simulink model "sine_kin"  (R2022a)
settings: Solver=VariableStepAuto  StartTime=0.0  StopTime=15  MaxStep=0.05  RelTol=1e-3
libraries: simulink x2
settings Model: Creator=patri  LastModifiedBy=Mattia
settings SolverCC: MaxConsecutiveMinStep=2  ShapePreserveControl=EnableAll

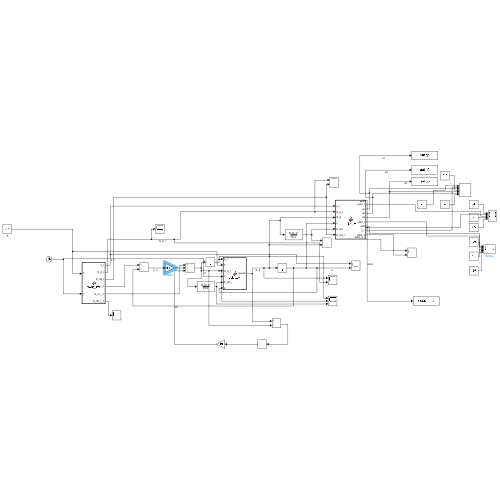
[thumbnail: Simulink's stored preview of the top-level diagram]
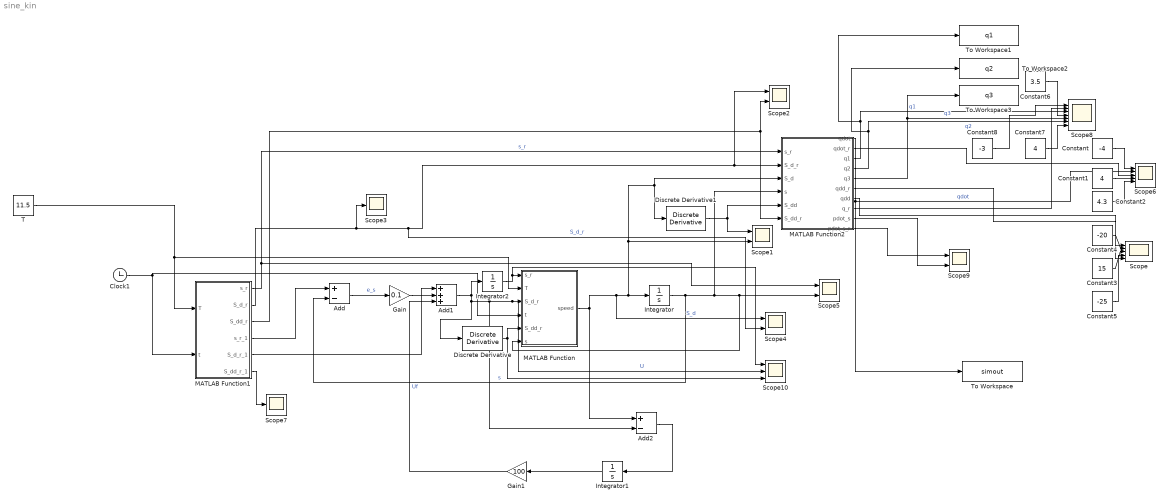
== system sine_kin ==
  Add : Sum  Inputs=+-
  Add1 : Sum  Inputs=+++
  Add2 : Sum  Inputs=+-
  Clock1 : Clock
  Constant : Constant  Value=-4
  Constant1 : Constant  Value=4
  Constant2 : Constant  Value=4.3
  Constant3 : Constant  Value=15
  Constant4 : Constant  Value=-20
  Constant5 : Constant  Value=-25
  Constant6 : Constant  Value=3.5
  Constant7 : Constant  Value=4
  Constant8 : Constant  Value=-3
  Discrete Derivative : simulink/Discrete/Discrete Derivative  gainval=1.0  ICPrevScaledInput=0.0  OutMin=[]  OutMax=[]  OutDataType=fixdt(1, 16)  OutScaling=2^-10  DoSatur=off
  Discrete Derivative1 : simulink/Discrete/Discrete Derivative  gainval=1.0  ICPrevScaledInput=0.0  OutMin=[]  OutMax=[]  OutDataType=fixdt(1, 16)  OutScaling=2^-10  DoSatur=off
  Gain : Gain  Gain=0.1
  Gain1 : Gain  Gain=100
  Integrator : Integrator
  Integrator1 : Integrator
  Integrator2 : Integrator
  MATLAB Function : MATLAB Function  TreatAsAtomicUnit=on
  MATLAB Function1 : MATLAB Function  TreatAsAtomicUnit=on
  MATLAB Function2 : MATLAB Function  TreatAsAtomicUnit=on
  Scope : Scope  NumInputPorts=5
  Scope{1..2,4..5,9} (5 alike) : Scope  NumInputPorts=2
  Scope10 : Scope  NumInputPorts=3
  Scope3 : Scope
  Scope6 : Scope  NumInputPorts=5
  Scope7 : Scope
  Scope8 : Scope  NumInputPorts=7
  T : Constant  Value=11.5
  To Workspace : ToWorkspace  VariableName=simout  SampleTime=-1
  To Workspace1 : ToWorkspace  VariableName=q1  SampleTime=-1
  To Workspace2 : ToWorkspace  VariableName=q2  SampleTime=-1
  To Workspace3 : ToWorkspace  VariableName=q3  SampleTime=-1
  wires:
  MATLAB Function1/1(s_r) -> MATLAB Function2/1(s_r), Scope5/1  "s_r"
  Add/1 -> Gain/1  "e_s"
  MATLAB Function1/2(S_d_r) -> Scope3/1, Scope4/2, Scope2/1, MATLAB Function2/2(S_d_r)  "S_d_r"
  Gain/1 -> Add1/2
  Add1/1 -> Discrete Derivative/1, Add2/2, Scope10/2, MATLAB Function/3(S_d_r), Integrator2/1  "U"
  MATLAB Function/1(speed) -> Scope4/1, Discrete Derivative1/1, MATLAB Function2/3(S_d), Scope1/2, Integrator/1, Add2/1  "S_d"
  Add2/1 -> Integrator1/1
  Integrator1/1 -> Gain1/1
  Gain1/1 -> Add1/3  "Uf"
  Integrator/1 -> Add/2, MATLAB Function2/4(s), MATLAB Function/6(s), Scope5/2  "s"
  Clock1/1 -> MATLAB Function1/2(t), MATLAB Function/4(t)
  MATLAB Function2/1(qdot) -> To Workspace/1, Scope6/2  "qdot"
  MATLAB Function2/2(qdot_r) -> Scope6/3
  MATLAB Function2/3(q1) -> To Workspace1/1, Scope8/3  "q1"
  MATLAB Function2/4(q2) -> To Workspace2/1, Scope8/6  "q2"
  MATLAB Function2/5(q3) -> To Workspace3/1, Scope8/5  "q3"
  T/1 -> MATLAB Function/2(T), MATLAB Function1/1(T)
  MATLAB Function2/6(qdd_r) -> Scope/1
  MATLAB Function2/7(qdd) -> Scope/5
  Constant/1 -> Scope6/1
  Constant1/1 -> Scope6/4
  Constant2/1 -> Scope6/5
  Constant5/1 -> Scope/4
  Constant3/1 -> Scope/3
  Discrete Derivative1/1 -> MATLAB Function2/5(S_dd), Scope1/1
  Constant4/1 -> Scope/2
  MATLAB Function1/3(S_dd_r) -> Scope2/2, MATLAB Function2/6(S_dd_r)
  MATLAB Function2/8(q_r) -> Scope8/2
  Constant6/1 -> Scope8/4
  Constant7/1 -> Scope8/7
  MATLAB Function2/9(pdot_s) -> Scope9/2
  MATLAB Function2/10(pdot_s_r) -> Scope9/1
  MATLAB Function1/4(s_r_1) -> Add/1
  MATLAB Function1/5(S_d_r_1) -> Add1/1
  MATLAB Function1/6(S_dd_r_1) -> Scope7/1
  Integrator2/1 -> Scope10/1, MATLAB Function/1(s_r)
  Discrete Derivative/1 -> Scope10/3, MATLAB Function/5(S_dd_r)
  Constant8/1 -> Scope8/1

== matlab function sine_kin/MATLAB Function ==
  data: s_r input; T input; speed output; S_d_r input; t input; S_dd_r input; s input
function speed = trajectory(s_r, T, S_d_r,t, S_dd_r, s)

%Links length
l1 = 1; l2 =1; l3 = 1;

%Trajectory


%%% REFERENCE


p_s_r =  [s_r + 1;
    1 + sin(4*pi*s_r);
    s_r];

R1_s_r=[1;
        4*pi*cos(4*pi*s_r);
        1];

%Velocity of the trajectory


%%pdot = R'*s'(t)




%%% REFERENCE

%%%POLYNOMIAL OF DEGREE 5 ---  0.4808 saturation --- 3.9 seconds
% pdot_s_r=[ -(30*t^2*pi*sin((2*t^3*pi*(10*T^2 - 15*T*t + 6*t^2))/T^5)*(T - t)^2)/T^5;
%           (30*t^2*pi*cos((2*t^3*pi*(10*T^2 - 15*T*t + 6*t^2))/T^5)*(T - t)^2)/T^5;
%                                                                                 0];
pdot_s_r= R1_s_r* S_d_r ; %sdr is u
      

%%%%%%%%%%%%%%%%%%%
% pdot_s_r = [-pi*sin(2*pi*((10*t^3)/T^3 - (15*t^4)/T^4 + (6*t^5)/T^5))*((30*t^2)/T^3 - (60*t^3)/T^4 + (30*t^4)/T^5);
%  pi*cos(2*pi*((10*t^3)/T^3 - (15*t^4)/T^4 + (6*t^5)/T^5))*((30*t^2)/T^3 - (60*t^3)/T^4 + (30*t^4)/T^5);
%                                                                                                      0];

%End effector position

%%% REFERENCE

px_r=p_s_r(1); py_r = p_s_r(2);
phi_r = p_s_r(3);

%%Inverse kinematics of planar 3R, compute q

%%% REFERENCE

p2_r = [px_r; py_r] - [l3*cos(phi_r); l3*sin(phi_r)];
p2x_r = p2_r(1);
p2y_r = p2_r(2);

% second joint computations


%%% REFERENCE

c2_r=(p2x_r^2+p2y_r^2-l1^2-l2^2)/(2*l1*l2); s2pos_r=sqrt(1-c2_r^2);

%other solution: -sqrt(1-c2^2)

%%% REFERENCE

s2neg_r=-sqrt(1-c2_r^2);

q02p_r=atan2(s2pos_r,c2_r);
q02n_r=atan2(s2neg_r,c2_r);
 
% first joint computations


%%% REFERENCE

detM_r=l1^2+l2^2+2*l1*l2*c2_r;

% positive solution of q1


%%% REFERENCE

s1pos_r=(p2y_r*(l1+l2*c2_r)-p2x_r*l2*s2pos_r)/detM_r; c1pos_r=(p2x_r*(l1+l2*c2_r)+p2y_r*l2*s2pos_r)/detM_r;

% negative solution of q1


%%% REFERENCE

s1neg_r=(p2y_r*(l1+l2*c2_r)-p2x_r*l2*s2neg_r)/detM_r;
c1neg_r=(p2x_r*(l1+l2*c2_r)+p2y_r*l2*s2neg_r)/detM_r;

q01p_r=atan2(s1pos_r,c1pos_r);
q01n_r=atan2(s1neg_r,c1neg_r); 

q03p_r = phi_r-(q01p_r+q02p_r);
q03n_r = phi_r-(q01n_r+q02n_r);



%%% REFERENCE


% output negative


%%% REFERENCE

q0n_r=[q01n_r; q02n_r; q03n_r];
q1_r = q0n_r(1);
q2_r = q0n_r(2);
q3_r = q0n_r(3);

%NOW WE COMPUTE qdot, qdotdot

%%% REFERENCE


P_r = [l1*cos(q1_r) + l2*cos(q1_r+q2_r) + l3*cos(q1_r+q2_r+q3_r);
    l1*sin(q1_r) + l2*sin(q1_r+q2_r) + l3*sin(q1_r+q2_r+q3_r)
    q1_r + q2_r + q3_r];

J_r = [- sin(q1_r + q2_r + q3_r) - sin(q1_r + q2_r) - sin(q1_r), - sin(q1_r + q2_r + q3_r) - sin(q1_r + q2_r), -sin(q1_r + q2_r + q3_r);
  cos(q1_r + q2_r + q3_r) + cos(q1_r + q2_r) + cos(q1_r),   cos(q1_r + q2_r + q3_r) + cos(q1_r + q2_r),  cos(q1_r + q2_r + q3_r);
                                          1,                                  1,                  1];


qdot_r = pinv(J_r) * pdot_s_r;

dq1_r=qdot_r(1);
dq2_r=qdot_r(2);
dq3_r=qdot_r(3);
J_dot_r = [- cos(q1_r + q2_r + q3_r)*(dq1_r + dq2_r + dq3_r) - cos(q1_r + q2_r)*(dq1_r + dq2_r) - dq1_r*cos(q1_r), - cos(q1_r + q2_r + q3_r)*(dq1_r + dq2_r + dq3_r) - cos(q1_r + q2_r)*(dq1_r + dq2_r), -cos(q1_r + q2_r + q3_r)*(dq1_r + dq2_r + dq3_r);
           - sin(q1_r + q2_r + q3_r)*(dq1_r + dq2_r + dq3_r) - sin(q1_r + q2_r)*(dq1_r + dq2_r) - dq1_r*sin(q1_r), - sin(q1_r + q2_r + q3_r)*(dq1_r + dq2_r + dq3_r) - sin(q1_r + q2_r)*(dq1_r + dq2_r), -sin(q1_r + q2_r + q3_r)*(dq1_r + dq2_r + dq3_r) ;   
            0,0,0];

%directly calculated
% pdd_r = [pi*sin(2*pi*((10*t^3)/T^3 - (15*t^4)/T^4 + (6*t^5)/T^5))*((60*t)/T^3 - (180*t^2)/T^4 + (120*t^3)/T^5) - 2*pi^2*cos(2*pi*((10*t^3)/T^3 - (15*t^4)/T^4 + (6*t^5)/T^5))*((30*t^2)/T^3 - (60*t^3)/T^4 + (30*t^4)/T^5)^2;
%        pi*cos(2*pi*((10*t^3)/T^3 - (15*t^4)/T^4 + (6*t^5)/T^5))*((60*t)/T^3 - (180*t^2)/T^4 + (120*t^3)/T^5) - 2*pi^2*sin(2*pi*((10*t^3)/T^3 - (15*t^4)/T^4 + (6*t^5)/T^5))*((30*t^2)/T^3 - (60*t^3)/T^4 + (30*t^4)/T^5)^2;
%         0];
 %%(60*t)/T^3 - (180*t^2)/T^4 + (120*t^3)/T^5

q1d_r=dq1_r;
q2d_r=dq2_r;
q3d_r=dq3_r;

pdotdot_s_r =[   0
        -16*pi^2*sin(4*pi*s_r)
                     0];

pdd_r = R1_s_r * S_dd_r + pdotdot_s_r * S_d_r^2;

qdd_r = inv(J_r)*(pdd_r - J_dot_r*qdot_r);

q1dd_r=qdd_r(1);
q2dd_r=qdd_r(2);
q3dd_r=qdd_r(3);
%%%%%%%%%%%%%%%%%%%%%%%%%%%%%%%%%%%%%%%%%%%%%%%%%%%%%%%%%%%%
%%bounds
q1_max=3.5;   q1_min=-3.5;
q2_max=3;     q2_min=-3;
q3_max= 2.57; q2_min =-2.57;
q1d_max= 4;   q1d_min=-4;
q2d_max=4;    q2d_min = -4;
q3d_max=4.3;  q3d_min=-4.3;
q1dd_max=20;  q1dd_min=-20;
q2dd_max=15;  q2dd_min=-15;
q3dd_max=20;  q3dd_min=-20;


constraint_pos = max([abs(q1_r/q1_max); abs(q2_r/q2_max);abs(q3_r/q3_max)]);

constraint_vel = max([abs(q1d_r/q1d_max);abs(q2d_r/q2d_max);abs(q3d_r/q3d_max)]);

constraint_acc = max([abs(q1dd_r/q1dd_max); abs(q2dd_r/q2dd_max);abs(q3dd_r/q3dd_max)]);

most_constrained = max([1;constraint_vel;(constraint_acc)]);

speed = S_d_r / most_constrained;

== matlab function sine_kin/MATLAB Function1 ==
  data: T input; t input; s_r output; S_d_r output; S_dd_r output; s_r_1 output; S_d_r_1 output; S_dd_r_1 output
function [s_r, S_d_r, S_dd_r,s_r_1, S_d_r_1, S_dd_r_1] = timing_law(T, t)
if t <T
    tau_t=t/T;
    %s_r = -2*tau_t^3 + 3*tau_t^2;
    %S_d_r=(6*t)/T^2 - (6*t^2)/T^3;
    s_r = 10*tau_t^3 - 15*tau_t^4 + 6*tau_t^5;
    S_d_r = (30*t^2)/T^3 - (60*t^3)/T^4 + (30*t^4)/T^5;
    S_dd_r = (60*t)/T^3 - (180*t^2)/T^4 + (120*t^3)/T^5;

    t_1 = t +0.0001;
    tau_t_1 = t_1/T;
    s_r_1 = 10*tau_t_1^3 - 15*tau_t_1^4 + 6*tau_t_1^5;
    S_d_r_1 = (30*t_1^2)/T^3 - (60*t_1^3)/T^4 + (30*t_1^4)/T^5;
    S_dd_r_1=(60*t_1)/T^3 - (180*t_1^2)/T^4 + (120*t_1^3)/T^5;

else 
    s_r = 1;
    S_d_r = 0;
    S_dd_r = 0;
    s_r_1 = 1;
    S_d_r_1 = 0;
    S_dd_r_1 = 0;
end

== matlab function sine_kin/MATLAB Function2 ==
  data: s_r input; S_d_r input; S_d input; s input; S_dd input; S_dd_r input; qdot output; qdot_r output; q1 output; q2 output; q3 output; qdd_r output; qdd output; q_r output; pdot_s output; pdot_s_r output
function [qdot,qdot_r,q1,q2,q3, qdd_r, qdd, q_r, pdot_s, pdot_s_r] = trajectory(s_r, S_d_r, S_d, s, S_dd, S_dd_r)

%Links length
l1 = 1; l2 =1; l3 = 1;

%Trajectory

p_s = [s + 1;
    1 + sin(4*pi*s);
    s];

p_s_r =  [s_r + 1;
    1 + sin(4*pi*s_r);
    s_r];

p1_s=[1;
        4*pi*cos(4*pi*s);
        1];
p1_s_r=[1;
        4*pi*cos(4*pi*s_r);
        1];

pdot_s= p1_s* S_d ;

                                                             
pdot_s_r = p1_s_r * S_d_r;
                                                             
                                                                    
%%%%%%%%%%%%%%%%%%%%%%%%%%%%%%%%%%%%%%%%%%%%%%%%%%%%%%%%%%%%%%%%
px = p_s(1); py = p_s(2); %position of the end effector w.r.t. the global frame

phi = p_s(3); %orientation of the end effector w.r.t. global frame

%%% REFERENCE

px_r=p_s_r(1); py_r = p_s_r(2);
phi_r = p_s_r(3);

%%Inverse kinematics of planar 3R
%fprintf("we first solve the joint variables q1, q2 in order to place\nthe position of the base of the third link in the necessary position\n");
 
p2 = [px; py] - [l3*cos(phi); l3*sin(phi)];
p2x = p2(1);
p2y = p2(2);

%%% REFERENCE

p2_r = [px_r; py_r] - [l3*cos(phi_r); l3*sin(phi_r)];
p2x_r = p2_r(1);
p2y_r = p2_r(2);

% second joint computations
c2=(p2x^2+p2y^2-l1^2-l2^2)/(2*l1*l2); 

%%% REFERENCE

c2_r=(p2x_r^2+p2y_r^2-l1^2-l2^2)/(2*l1*l2);

%other solution: -sqrt(1-c2^2)
s2neg=-sqrt(1-c2^2);


q02n=atan2(s2neg,c2);

%%% REFERENCE

s2neg_r=-sqrt(1-c2_r^2);


q02n_r=atan2(s2neg_r,c2_r);
 
% first joint computations
detM=l1^2+l2^2+2*l1*l2*c2;

%%% REFERENCE

detM_r=l1^2+l2^2+2*l1*l2*c2_r;


%%% REFERENCE



% negative solution of q1
s1neg=(p2y*(l1+l2*c2)-p2x*l2*s2neg)/detM;
c1neg=(p2x*(l1+l2*c2)+p2y*l2*s2neg)/detM;

q01n=atan2(s1neg,c1neg);
q03n = phi-(q01n+q02n);

%%% REFERENCE

s1neg_r=(p2y_r*(l1+l2*c2_r)-p2x_r*l2*s2neg_r)/detM_r;
c1neg_r=(p2x_r*(l1+l2*c2_r)+p2y_r*l2*s2neg_r)/detM_r;


q01n_r=atan2(s1neg_r,c1neg_r); 

q03n_r = phi_r-(q01n_r+q02n_r);


%%% REFERENCE


% output negative
q0n=[q01n; q02n; q03n];

%%% REFERENCE

q0n_r=[q01n_r; q02n_r; q03n_r];
q_r = q0n_r;
%In a cubic polynomial the maximum of the speed of the timing law is
%obtained in t = T/2 
q1 = q0n(1);
q2 = q0n(2);
q3 = q0n(3);
P = [l1*cos(q1) + l2*cos(q1+q2) + l3*cos(q1+q2+q3);
    l1*sin(q1) + l2*sin(q1+q2) + l3*sin(q1+q2+q3)
    q1 + q2 + q3];

J = [- sin(q1 + q2 + q3) - sin(q1 + q2) - sin(q1), - sin(q1 + q2 + q3) - sin(q1 + q2), -sin(q1 + q2 + q3);
  cos(q1 + q2 + q3) + cos(q1 + q2) + cos(q1),   cos(q1 + q2 + q3) + cos(q1 + q2),  cos(q1 + q2 + q3);
                                          1,                                  1,                  1];

%%% REFERENCE

q1_r = q0n_r(1);
q2_r = q0n_r(2);
q3_r = q0n_r(3);

P_r = [l1*cos(q1_r) + l2*cos(q1_r+q2_r) + l3*cos(q1_r+q2_r+q3_r);
    l1*sin(q1_r) + l2*sin(q1_r+q2_r) + l3*sin(q1_r+q2_r+q3_r)
    q1 + q2 + q3];

J_r = [- sin(q1_r + q2_r + q3_r) - sin(q1_r + q2_r) - sin(q1_r), - sin(q1_r + q2_r + q3_r) - sin(q1_r + q2_r), -sin(q1_r + q2_r + q3_r);
  cos(q1_r + q2_r + q3_r) + cos(q1_r + q2_r) + cos(q1_r),   cos(q1_r + q2_r + q3_r) + cos(q1_r + q2_r),  cos(q1_r + q2_r + q3_r);
                                          1,                                  1,                  1];


qdot = pinv(J) * pdot_s;
dq1 = qdot(1);
dq2 = qdot(2);
dq3 = qdot(3);

p2_s =[   0
-16*pi^2*sin(4*pi*s)
                     0];

J_dot = [- cos(q1 + q2 + q3)*(dq1 + dq2 + dq3) - cos(q1 + q2)*(dq1 + dq2) - dq1*cos(q1), - cos(q1 + q2 + q3)*(dq1 + dq2 + dq3) - cos(q1 + q2)*(dq1 + dq2), -cos(q1 + q2 + q3)*(dq1 + dq2 + dq3);
    - sin(q1 + q2 + q3)*(dq1 + dq2 + dq3) - sin(q1 + q2)*(dq1 + dq2) - dq1*sin(q1), - sin(q1 + q2 + q3)*(dq1 + dq2 + dq3) - sin(q1 + q2)*(dq1 + dq2), -sin(q1 + q2 + q3)*(dq1 + dq2 + dq3);
    0,0,0];
pdd = p1_s * S_dd + p2_s * S_d^2;
qdd = inv(J)*(pdd - J_dot*qdot);
%%% REFERENCE

qdot_r = pinv(J_r) * pdot_s_r;

qdot = qdot;
dq1_r = qdot_r(1); dq2_r = qdot_r(2); dq3_r = qdot_r(3);
qdot_r = qdot_r;
J_dot_r = [- cos(q1_r + q2_r + q3_r)*(dq1_r + dq2_r + dq3_r) - cos(q1_r + q2_r)*(dq1_r + dq2_r) - dq1_r*cos(q1_r), - cos(q1_r + q2_r + q3_r)*(dq1_r + dq2_r + dq3_r) - cos(q1_r + q2_r)*(dq1_r + dq2_r), -cos(q1_r + q2_r + q3_r)*(dq1_r + dq2_r + dq3_r);
           - sin(q1_r + q2_r + q3_r)*(dq1_r + dq2_r + dq3_r) - sin(q1_r + q2_r)*(dq1_r + dq2_r) - dq1_r*sin(q1_r), - sin(q1_r + q2_r + q3_r)*(dq1_r + dq2_r + dq3_r) - sin(q1_r + q2_r)*(dq1_r + dq2_r), -sin(q1_r + q2_r + q3_r)*(dq1_r + dq2_r + dq3_r) ;   
            0,0,0];
%pdd_r =  [                                                                                                                                                                            (60*t)/T^3 - (180*t^2)/T^4 + (120*t^3)/T^5
%4*pi*cos(4*pi*((10*t^3)/T^3 - (15*t^4)/T^4 + (6*t^5)/T^5))*((60*t)/T^3 - (180*t^2)/T^4 + (120*t^3)/T^5) - 16*pi^2*sin(4*pi*((10*t^3)/T^3 - (15*t^4)/T^4 + (6*t^5)/T^5))*((30*t^2)/T^3 - (60*t^3)/T^4 + (30*t^4)/T^5)^2
%                                                                                                                                                                            (60*t)/T^3 - (180*t^2)/T^4 + (120*t^3)/T^5];
p2_s_r =[   0
-16*pi^2*sin(4*pi*s_r)
                     0];
pdd_r = p1_s_r * S_dd_r + p2_s_r * S_d_r^2;
qdd_r = inv(J_r)*(pdd_r - J_dot_r*qdot_r);
